simulink model "Pendulosimple"  (R2020b)
settings: Solver=VariableStepAuto  StartTime=0.0  StopTime=30  MaxStep=0.01  RelTol=1e-3
settings Model: Creator=User  LastModifiedBy=sofia
settings SFSimCC: CustomCodeUndefinedFunction=UseInterfaceOnly

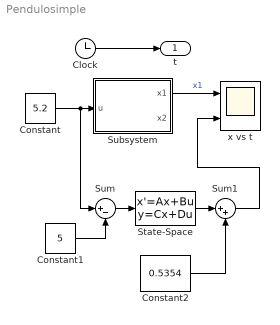
== system Pendulosimple ==
  Clock : Clock
  Constant : Constant  Value=5.2
  Constant1 : Constant  Value=5
  Constant2 : Constant  Value=0.5354
  State-Space : StateSpace  A=[0 1;-8.4290 -0.5]  B=[0;1]  C=[1 0]  D=0  InitialCondition=0.8-0.5354
  Subsystem : Subsystem  mask{m=1, g=9.81, l=1, f=0.5, ci=[0.8  0]}
      mask prompts: m "m(mass, Kg)"; g "g(gravity, m s^-2)"; l "l(lenght, m)"; f "f(fricction, N s m^-1)"; ci "c.i.[x10,x20]"
      mask init:
      | x10 = ci(1);
      | x20 = ci(2);
      mask DialogControl DescGroupVar Prompt: Pendulo simple
      mask DialogControl DescTextVar Prompt: N = Newton, s = Segundo, m = Metro, Kg = Kilogramo, x10= condicion inicial de x1 en radianes, x20= condicion inicial de x2 en radianes / s
      mask Display: disp('Sistema de \npéndulo simple')
  Sum : Sum  Inputs=|+-
  Sum1 : Sum  Inputs=|++
  x vs t : Scope  NumInputPorts=2
  t : Outport  VectorParamsAs1DForOutWhenUnconnected=off
  wires:
  Subsystem/1(x1) -> x vs t/1  "x1"
  Clock/1 -> t/1
  Constant/1 -> Sum/1, Subsystem/1(u)
  Sum/1 -> State-Space/1
  Constant1/1 -> Sum/2
  State-Space/1 -> Sum1/1
  Constant2/1 -> Sum1/2
  Sum1/1 -> x vs t/2

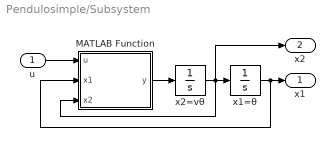
== system Pendulosimple/Subsystem ==
  u : Inport
  MATLAB Function : MATLAB Function  TreatAsAtomicUnit=on
  x1=θ : Integrator  InitialCondition=x10
  x2=vθ : Integrator  InitialCondition=x20
  x1 : Outport  VectorParamsAs1DForOutWhenUnconnected=off
  x2 : Outport  Port=2  VectorParamsAs1DForOutWhenUnconnected=off
  wires:
  u/1 -> MATLAB Function/1(u)
  MATLAB Function/1(y) -> x2=vθ/1
  x1=θ/1 -> MATLAB Function/2(x1), x1/1
  x2=vθ/1 -> MATLAB Function/3(x2), x2/1, x1=θ/1

== matlab function Pendulosimple/Subsystem/MATLAB Function ==
  data: u input; x1 input; x2 input; y output; g parameter; l parameter; f parameter; m parameter
function y = fcn(u,x1,x2,g, l, f, m)
y = -((g/l)*sin(x1))-((f/m)*x2)+(u/(m*l));
